simulink library "sm_car_scene_rdf_rough_road"  (R2025a)
settings: Solver=VariableStepAuto  StartTime=0.0  StopTime=10.0  RelTol=1e-3
undefined symbols (not defined in the file or in its folder): Scene
libraries: Scene_Utilities x1
Description:
  | Scene of Simscape Vehicle Templates Library
  | 
  | Copyright 2018-2025 The MathWorks, Inc.
settings Model: Creator=smiller  LastModifiedBy=smiller
settings SolverCC: AlgebraicLoopSolver=TrustRegion
settings DataIOCC: ReturnWorkspaceOutputs=off
settings OptimizationCC: ReuseModelBlockBuffer=off
settings DebuggingCC: UnconnectedInputMsg=warning  UnconnectedOutputMsg=warning  UnconnectedLineMsg=warning  ArithmeticOperatorsInVariantConditions=warning
settings ModelReferenceCC: EnableRefExpFcnMdlSchedulingChecks=on
settings SFSimCC: CustomCodeUndefinedFunction=UseInterfaceOnly
settings RTWCC: GPUComputeCapability=3.5  DLArmComputeVersion=19.05

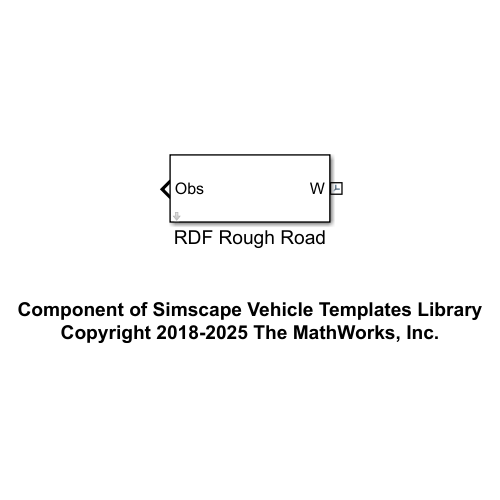
[thumbnail: Simulink's stored preview of the top-level diagram]
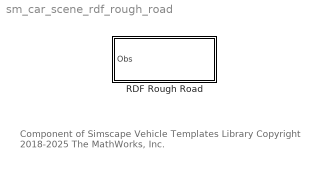
== system sm_car_scene_rdf_rough_road ==
  note: Component of Simscape Vehicle Templates Library
      | Copyright 2018-2025 The MathWorks, Inc.
  RDF Rough Road : Subsystem  mask{RDF_Polyline=Scene.RDF_Rough_Road}
      mask prompts: RDF_Polyline "RDF Polyline (structure)"

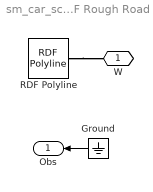
== system sm_car_scene_rdf_rough_road/RDF Rough Road ==
  Ground : Ground
  RDF Polyline : Scene_Utilities/RDF Polyline  road_extr_data_L=RDF_Polyline.Road.extr_data_L  road_extr_data_R=RDF_Polyline.Road.extr_data_R  road_profile_sep=RDF_Polyline.Road.profile_separation  road_w=RDF_Polyline.Road.w  road_x=RDF_Polyline.Road.x  road_z=RDF_Polyline.Road.z  road_yaw=RDF_Polyline.Road.yaw  road_clr=RDF_Polyline.Road.clr  road_opc=RDF_Polyline.Road.opc
  W : PMIOPort  Side=Left
  Obs : Outport  VectorParamsAs1DForOutWhenUnconnected=off
  wires:
  Ground/1 -> Obs/1
  connections:
  RDF Polyline/RConn1 -- W/RConn1
